simulink model "SVL_VV_PIDschema"  (R2018b)
settings: Solver=VariableStepAuto  StartTime=0.0  StopTime=3.6295  FixedStep=0.01  RelTol=1e-5
settings Model: Creator=Marek  LastModifiedBy=Marek

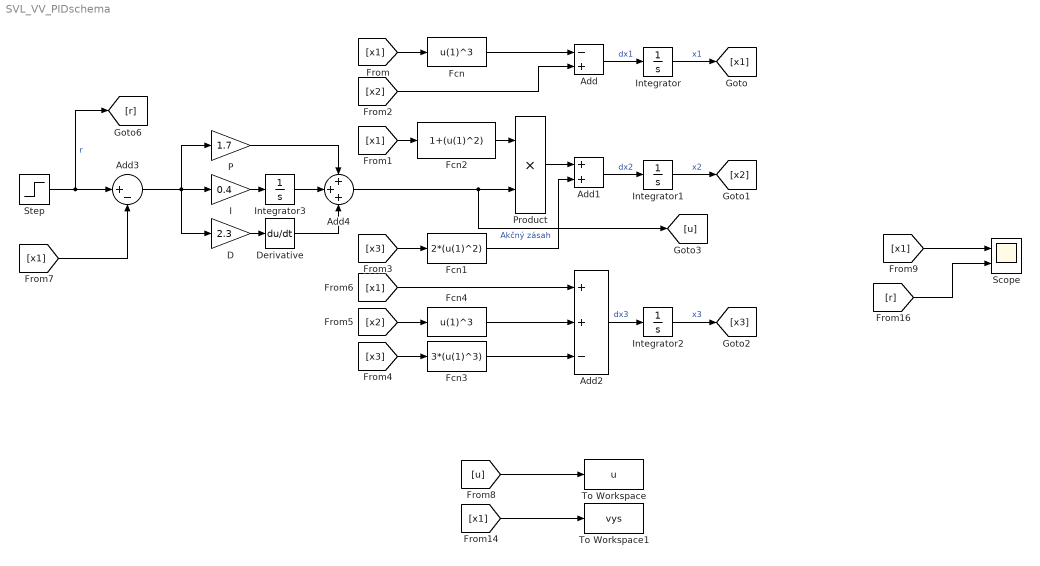
== system SVL_VV_PIDschema ==
  Add : Sum  Inputs=-+
  Add1 : Sum
  Add2 : Sum  Inputs=++-
  Add3 : Sum  Inputs=|+-
  Add4 : Sum  Inputs=+++
  D : Gain  Gain=2.3
  Derivative : Derivative
  Fcn : Fcn  Expr=u(1)^3
  Fcn1 : Fcn  Expr=2*(u(1)^2)
  Fcn2 : Fcn  Expr=1+(u(1)^2)
  Fcn3 : Fcn  Expr=3*(u(1)^3)
  Fcn4 : Fcn  Expr=u(1)^3
  I : Gain  Gain=0.4
  Integrator{,1..3} (4 alike) : Integrator
  P : Gain  Gain=1.7
  Product : Product
  Scope : Scope  NumInputPorts=2
  Step : Step  Time=0  After=-1  SampleTime=0
  To Workspace : ToWorkspace  VariableName=u  SaveFormat=Timeseries  SampleTime=-1
  To Workspace1 : ToWorkspace  VariableName=vys  SaveFormat=Timeseries  SampleTime=-1
  wires:
  [r] -> Scope/2
  Add/1 -> Integrator/1  "dx1"
  Integrator1/1 -> [x2]  "x2"
  Add1/1 -> Integrator1/1  "dx2"
  Fcn2/1 -> Product/1
  [x2] -> Add/2
  Integrator2/1 -> [x3]  "x3"
  Integrator/1 -> [x1]  "x1"
  Fcn/1 -> Add/1
  Fcn1/1 -> Add1/2
  [x3] -> Fcn3/1
  Add2/1 -> Integrator2/1  "dx3"
  Step/1 -> [r], Add3/1  "r"
  Fcn3/1 -> Add2/3
  [x1] -> Add2/1
  [x1] -> Fcn2/1
  [x2] -> Fcn4/1
  Fcn4/1 -> Add2/2
  [x3] -> Fcn1/1
  [x1] -> Fcn/1
  Product/1 -> Add1/1
  [x1] -> Add3/2
  Add3/1 -> D/1, I/1, P/1
  D/1 -> Derivative/1
  I/1 -> Integrator3/1
  Integrator3/1 -> Add4/2
  Derivative/1 -> Add4/3
  P/1 -> Add4/1
  Add4/1 -> [u], Product/2  "Akčný zásah"
  [u] -> To Workspace/1
  [x1] -> To Workspace1/1
  [x1] -> Scope/1
